simulink model "SimScape_PSFB_PCMC_HalfBridge_SRMode0"  (R2023b)
settings: Solver=VariableStepAuto  StartTime=0.0  StopTime=0.5  RelTol=1e-3
undefined symbols (not defined in the file): ADC_MaxCount, ADC_Vref, Gi_fb, L, Lm, n, Rload, Ro, Tcmpss, transformerCoupling
libraries: ee_lib x15, fl_lib x14, nesl_utility x9, simulink_extras x2, simulink x2, slpidlib x1
(part 1 of 2)
settings Model: Creator=a0485298  LastModifiedBy=a0485298

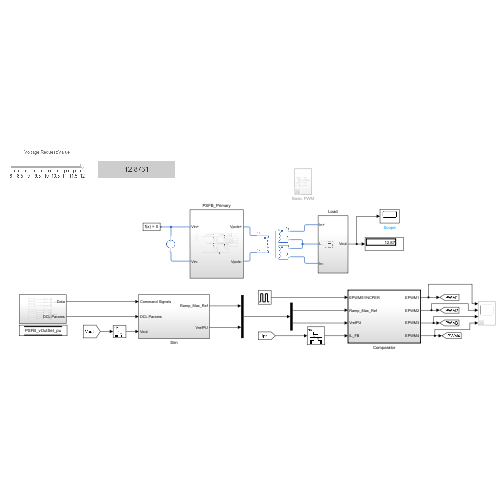
[thumbnail: Simulink's stored preview of the top-level diagram]
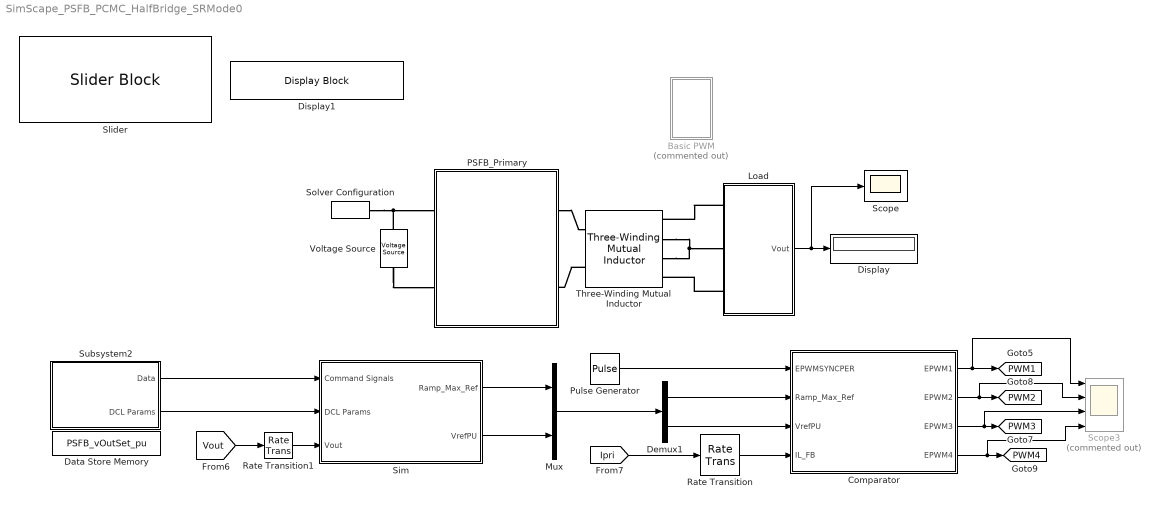
== system SimScape_PSFB_PCMC_HalfBridge_SRMode0 ==
  Basic PWM : Subsystem  Commented=on
  Comparator : Subsystem  TreatAsAtomicUnit=on
  Data Store Memory : DataStoreMemory  DataStoreName=PSFB_vOutSet_pu  WriteAfterWriteMsg=warning  ShowAdditionalParam=off
  Demux1 : Demux  Outputs=2
  Display : Display
  Display1 : DisplayBlock  LabelPosition=Hide  Transparency=1
  Load : Subsystem
      settings: PortSchema="{\"entries\":[{\"content\":{\"sides\":[{\"content\":{\"connectorIds\":[\"Out1\"]},\"type\":\"ConnectorPlacement.EquallySpacedRectSide\",\"uuid\":\"d456934f-8cdc-4057-8992-94e9047cf07f\"},{\"content\":{\"connectorIds\":[\"RConn1\",\"RConn2\",\"RConn3\"],\"side\":\"RIGHT\"},\"type\":\"ConnectorPlacement.EquallySpacedRectSide\",\"uuid\":\"13bc9f8f-848a-4da9-bcdd-c680aa1b8ed2\"},{\"content\":{\"side\":\"TOP\"},\"type\":\"ConnectorPlacement.EquallySpacedRectSide\",\"uuid\":\"cb883331-c911-4e56-96a8-3c5b8591d015\"}]},\"type\":\"ConnectorPlacement.EquallySpacedConnector\",\"uuid\":\"df461162-389f-468c-a658-0242576d1be7\"}],\"packageUris\":[\"http://schema.mathworks.com/mf0/Connector/R2020b\"],\"version\":\"1.0\"}"
  Mux : Mux  Inputs=2
  PSFB_Primary : Subsystem
  Pulse Generator : DiscretePulseGenerator  PulseType=Time based  Period=1/200e3  PulseWidth=5
  Rate Transition : RateTransition
  Rate Transition1 : RateTransition
  Scope : Scope
  Scope3 : Scope  Commented=on  NumInputPorts=4
  Sim : Subsystem  RTWFileName=sample_cla  VariantControl=(sim)
      settings: RTWSystemCode=Nonreusable function  RTWFileNameOpts=User specified  FunctionWithSeparateData=on  RTWMemSecFuncInitTerm=C28xFunction  RTWMemSecFuncExecute=ClaFunction  RTWMemSecDataConstants=Cla1DataRam  RTWMemSecDataInternal=Cla1DataRam  RTWMemSecDataParameters=Cla1DataRam
  Slider : SliderBlock  ScaleMin=8  ScaleMax=12  TickInterval=0.5
  Solver Configuration : nesl_utility/Solver Configuration  PhysicalDomain=network_engine_domain  SubClassName=solver  LeftPortType=input  RightPortType=generic  Tones=[]  Harmonics=[]  SimulateNoise=off  Profile=off  UseLocalSampling=off  EnableSwitchedLinearOptims=on  FrequencyDomain=off  UseCCode=off  RelTol=0.001  AbsTol=0.001  MinStep=1e-09  ToWorkspace=off  RevertToSquareIcSolve=off  NumHomotopyIterations=100  PhasorMode=off  PhasorModeNumHarmonics=1  ConsistencySolver=NEWTON_XTOL_AFTER_FTOL  IndexReductionMethod=DerivativeReplacement  DoDC=off  ResidualTolerance=1e-09  ConsistencyTolSource=GLOBAL  ConsistencyAbsTol=0.001  ConsistencyRelTol=0.001  ConsistencyTolFactor=0.001  UseLocalSolver=on  LocalSolverChoice=NE_BACKWARD_EULER_ADVANCER  ResolveIndetEquations=on  FunctionEvalNumThread=1  LocalSolverSampleTime=1/120e6  DoFixedCost=off  MaxNonlinIter=3  MaxModeIter=2  ComputeImpulses=off  ImpulseIterations=2  LinearAlgebra=auto  LinearAlgebraNumThread=0  EquationFormulation=NE_TIME_EF  DelaysMemoryBudget=1024  AutomaticFiltering=off  FilteringTimeConstant=0.001  PartitionStorageMethod=AS_NEEDED  PartitionMemoryBudget=1024  PartitionMethod=ROBUST  MultibodyUseLocalSolver=off  MultibodyLocalSolverChoice=ODE1  MultibodyLocalSolverSampleTime=0.001
  Subsystem2 : Subsystem
  Three-Winding Mutual Inductor : ee_lib/Passive/Transformers/Three-Winding Mutual Inductor  L1=Lm/transformerCoupling^2 H  L2=Lm/n^2 H  L3=Lm/n^2 H  K12=transformerCoupling  K13=transformerCoupling  K23=transformerCoupling  IC_given=1  IC1=0 A  IC2=0 A  IC3=0 A
      settings: InternalSimscapePortConfiguration="{\"Bottom\":[],\"Left\":[{\"id\":\"p1\",\"label\":\"1+\",\"type\":\"foundation.electrical.electrical\"},{\"id\":\"n1\",\"label\":\"1-\",\"type\":\"foundation.electrical.electrical\"}],\"Right\":[{\"id\":\"p2\",\"label\":\"2+\",\"type\":\"foundation.electrical.electrical\"},{\"id\":\"n2\",\"label\":\"2-\",\"type\":\"foundation.electrical.electrical\"},{\"id\":\"p3\",\"label\":\"3+\",\"type\":\"foundation.electrical.electrical\"},{\"id\":\"n3\",\"label\":\"3-\",\"type\":\"foundation.electrical.electrical\"}],\"Top\":[]}"
  Voltage Source : ee_lib/Sources/Voltage Source  dc_voltage=Vin V  ac_voltage=0 V  ac_shift=0 rad  ac_frequency=60 Hz  noise_mode=ee.enum.sources.noise.Disabled  PSD=0 V^2/Hz  sample_time=1e-3 s  repeatability=ee.enum.sources.repeatability.NotRepeatable  user_seed=0  auto_seed=3890346746  i_specify=off  i_priority=None  i=0 A  i_nominal_specify=off  i_nominal_unit=A  i_nominal_value=1  v_specify=off  v_priority=None  v=0 V  v_nominal_specify=off  v_nominal_unit=V  v_nominal_value=1
  tag scope: PWM1=global, PWM2=global, PWM3=global, PWM4=global
  wires:
  Load/1(Vout) -> Scope/1, Display/1
  Demux1/2 -> Comparator/3(VrefPU)
  Sim/1(Ramp_Max_Ref) -> Mux/1
  Mux/1 -> Demux1/1
  Comparator/2(EPWM2) -> Scope3/2, [PWM2]
  Subsystem2/2(DCL Params) -> Sim/2(DCL Params)
  [Vout] -> Rate Transition1/1
  Pulse Generator/1 -> Comparator/1(EPWMSYNCPER)
  Comparator/4(EPWM4) -> Scope3/4, [PWM4]
  Comparator/1(EPWM1) -> Scope3/1, [PWM1]
  Demux1/1 -> Comparator/2(Ramp_Max_Ref)
  Subsystem2/1(Data) -> Sim/1(Command Signals)
  Comparator/3(EPWM3) -> Scope3/3, [PWM3]
  Sim/2(VrefPU) -> Mux/2
  [Ipri] -> Rate Transition/1
  Rate Transition1/1 -> Sim/3(Vout)
  Rate Transition/1 -> Comparator/4(IL_FB)
  connections:
  Load/RConn3 -- Three-Winding Mutual Inductor/RConn4
  Three-Winding Mutual Inductor/RConn2 -- Three-Winding Mutual Inductor/RConn3 -- Load/RConn2
  Three-Winding Mutual Inductor/LConn2 -- PSFB_Primary/LConn2
  PSFB_Primary/LConn1 -- Three-Winding Mutual Inductor/LConn1
  Load/RConn1 -- Three-Winding Mutual Inductor/RConn1
  Voltage Source/LConn1 -- PSFB_Primary/RConn1 -- Solver Configuration/RConn1
  Voltage Source/RConn1 -- PSFB_Primary/RConn2

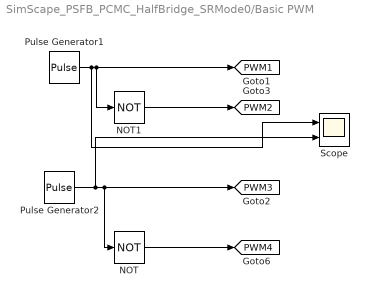
== system SimScape_PSFB_PCMC_HalfBridge_SRMode0/Basic PWM ==
  NOT : Logic  Operator=NOT  IconShape=distinctive  AllPortsSameDT=off  OutDataTypeStr=boolean
  NOT1 : Logic  Operator=NOT  IconShape=distinctive  AllPortsSameDT=off  OutDataTypeStr=boolean
  Pulse Generator1 : DiscretePulseGenerator  PulseType=Time based  Period=1/100e3  PulseWidth=50
  Pulse Generator2 : DiscretePulseGenerator  PulseType=Time based  Period=1/100e3  PulseWidth=50  PhaseDelay=(72/(180*100e3))
  Scope : Scope  NumInputPorts=2
  tag scope: PWM1=global, PWM2=global, PWM3=global, PWM4=global
  wires:
  Pulse Generator1/1 -> Scope/1, [PWM1], NOT1/1
  NOT1/1 -> [PWM2]
  Pulse Generator2/1 -> Scope/2, [PWM3], NOT/1
  NOT/1 -> [PWM4]

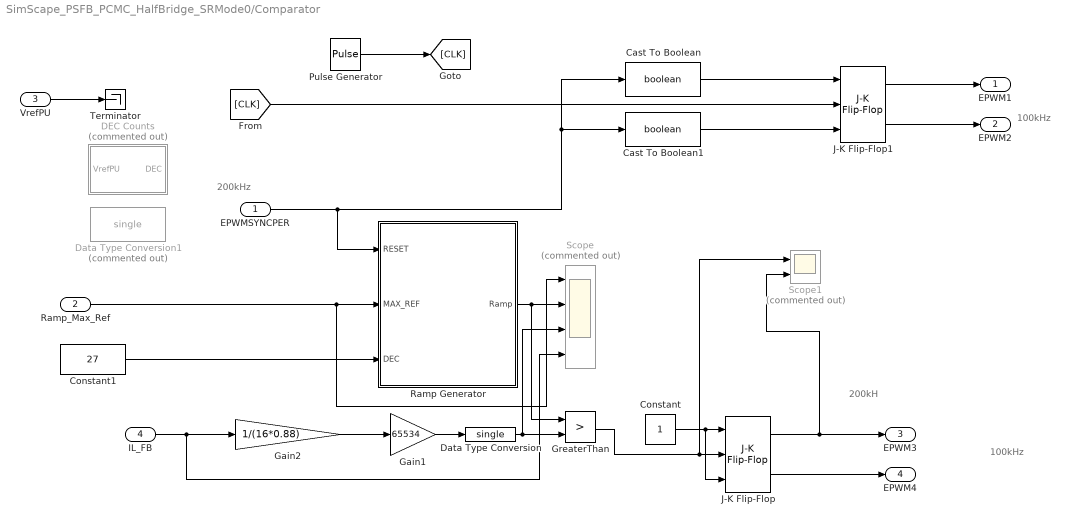
== system SimScape_PSFB_PCMC_HalfBridge_SRMode0/Comparator ==
  note: 200kH
  note: 100kHz
  note: 100kHz
  note: 200kHz
  EPWMSYNCPER : Inport
  Ramp_Max_Ref : Inport  Port=2
  VrefPU : Inport  Port=3
  IL_FB : Inport  Port=4
  Cast To Boolean : DataTypeConversion  OutDataTypeStr=boolean  SaturateOnIntegerOverflow=off  RndMeth=Floor
  Cast To Boolean1 : DataTypeConversion  OutDataTypeStr=boolean  SaturateOnIntegerOverflow=off  RndMeth=Floor
  Constant : Constant  OutDataTypeStr=boolean
  Constant1 : Constant  Value=27  OutDataTypeStr=single
  DEC Counts : Subsystem  Commented=on
  Data Type Conversion : DataTypeConversion  OutDataTypeStr=single  SaturateOnIntegerOverflow=off  RndMeth=Floor
  Data Type Conversion1 : DataTypeConversion  Commented=on  OutDataTypeStr=single  SaturateOnIntegerOverflow=off  RndMeth=Floor
  Gain1 : Gain  Gain=65534  OutDataTypeStr=single
  Gain2 : Gain  Gain=1/(16*0.88)  OutDataTypeStr=single
  GreaterThan : RelationalOperator  Operator=>  OutDataTypeStr=boolean  RndMeth=Simplest  InputSameDT=off
  J-K Flip-Flop : simulink_extras/Flip Flops/J-K Flip-Flop  initial_condition=0
  J-K Flip-Flop1 : simulink_extras/Flip Flops/J-K Flip-Flop  initial_condition=0
  Pulse Generator : DiscretePulseGenerator  PulseType=Time based  Period=1/(2*200e3)
  Ramp Generator : Subsystem
  Scope : Scope  Commented=on  NumInputPorts=4
  Scope1 : Scope  Commented=on  NumInputPorts=2
  Terminator : Terminator
  EPWM1 : Outport
  EPWM2 : Outport  Port=2
  EPWM3 : Outport  Port=3
  EPWM4 : Outport  Port=4
  wires:
  Gain2/1 -> Gain1/1
  IL_FB/1 -> Scope/4, Gain2/1
  EPWMSYNCPER/1 -> Cast To Boolean1/1, Cast To Boolean/1, Ramp Generator/1(RESET)
  Ramp Generator/1(Ramp) -> GreaterThan/1, Scope/2
  Gain1/1 -> Data Type Conversion/1
  J-K Flip-Flop/1 -> Scope1/2, EPWM3/1
  J-K Flip-Flop/2 -> EPWM4/1
  Pulse Generator/1 -> [CLK]
  [CLK] -> J-K Flip-Flop1/2
  J-K Flip-Flop1/1 -> EPWM1/1
  J-K Flip-Flop1/2 -> EPWM2/1
  Cast To Boolean/1 -> J-K Flip-Flop1/1
  Cast To Boolean1/1 -> J-K Flip-Flop1/3
  VrefPU/1 -> Terminator/1
  Constant1/1 -> Ramp Generator/3(DEC)
  Constant/1 -> J-K Flip-Flop/3, J-K Flip-Flop/1
  GreaterThan/1 -> Scope1/1, J-K Flip-Flop/2
  Ramp_Max_Ref/1 -> Scope/1, Ramp Generator/2(MAX_REF)
  Data Type Conversion/1 -> Scope/3, GreaterThan/2

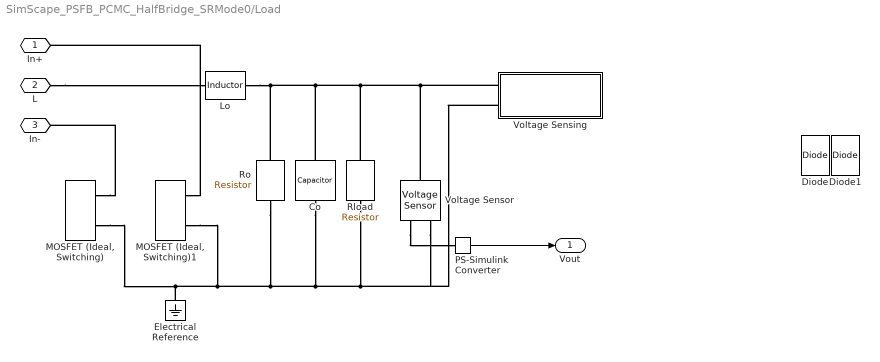
== system SimScape_PSFB_PCMC_HalfBridge_SRMode0/Load ==
  Co : fl_lib/Electrical/Electrical Elements/Capacitor  c=Co F  r=1e-6 Ohm  g=0 1/Ohm  i_specify=off  i_priority=None  i=0 A  i_nominal_specify=off  i_nominal_unit=A  i_nominal_value=1  v_specify=off  v_priority=None  v=0 V  v_nominal_specify=off  v_nominal_unit=V  v_nominal_value=30  vc_specify=off  vc_priority=High  vc=0 V  vc_nominal_specify=off  vc_nominal_unit=V  vc_nominal_value=1
  Diode : ee_lib/Semiconductors & Converters/Diode  ModelType=ee.enum.diode.modelType.pwl  TableType=ee.enum.diode.tableType.IfMat  IfMat=[.07, .12, .19, 1.75, 4.24, 7.32, 11.2; .16, .3, .72, 2.14, 5.02, 8.35, 13.12] A  VfMat=[.9, 1.15, 1.25, 1.5, 1.75, 2.17, 2.6, 2.85; .58, .68, .75, 1.1, 1.38, 1.77, 2.27, 2.7] V  TjVec=[25, 125] degC  VfVec=[.5, .7, .9, 1.3, 1.7, 2.1, 2.5] V  IfVec=[.1, .2, .5, 1, 2, 4, 7, 10] A  Vf=0.6 V  Ron=1e-6 Ohm  Goff=1e-8 S  prmExp=ee.enum.diode.expParam.useTwo  I12=[.0137, .545] A  V12=[.6, .7] V  RS=0 Ohm  Tmeas=25 degC  IS=1e-12 A  ec=1  I1=0.0137 A  V1=0.6 V  N_series=1  N_parallel=1  ZenerEnable=false  Rz=0.3 Ohm  BV=inf V  C_param=ee.enum.diode.capParam.fixed  CJ=0 pF  CJ0=5 pF  Vvec=[.1, 10, 100] V  Cvec=[3.5, 1, .4] pF  VJ=1 V  Mgrad=0.5  FC=0.5  Q_param=ee.enum.diode.recoveryParam.off  iRM=-7.15 A  iF=4 A  didt=-750 A/us  trr_factor=3  trr=115 ns  Qrr=150 nA*s  Vr=-600 V  Ls=150 nH  Erec=0.03 J  TT=50 ns  tau=100 ns  T_param=ee.enum.diode.temperatureParam.off  Tdevice=25 degC  I1_T2=0.245 A  V1_T2=0.5 V  IS_T2=1.25e-7 A  Tmeas2=125 degC  XTI_param=ee.enum.diode.xtiParam.pn  XTI=3  EG_param=ee.enum.diode.egapParam.material_si  EG=1.11 eV  dBVdT=0 V/K  enable_faults=simscape.enum.onoff.off  fault_action=simscape.enum.assert.action.none  fault_types=ee.enum.diode.faults.open  tau_fault=1e-3 s  IfMat_faulted=[.07, .12, .19, 1.75, 4.24, 7.32, 11.2; .16, .3, .72, 2.14, 4.02, 6.35, 9.12] A  VfMat_faulted=[.9, 1.15, 1.25, 1.5, 1.75, 2.17, 2.6, 2.85; .58, .68, .75, 1.1, 1.38, 1.77, 2.27, 2.7] V  VfVec_faulted=[.5, .7, .9, 1.3, 1.7, 2.1, 2.5] V  IfVec_faulted=[.1, .2, .5, 1, 2, 4, 7, 10] A  Ropen_faulted=1000 Ohm  Gshort_faulted=1000 1/Ohm  Vf_faulted=0.6 V  Ron_faulted=0.3 Ohm  Goff_faulted=1e-8 S  I12_faulted=[.0137, .545] A  V12_faulted=[.6, .7] V  IS_faulted=1e-12 A  ec_faulted=1  I1_faulted=0.0137 A  V1_faulted=0.6 V  RS_faulted=0 Ohm  Rz_faulted=0.3 Ohm  BV_faulted=inf V  Cscale_faulted=100  fault_trigger=ee.enum.faults.faultTrigger.temporal  t_fault=inf s  max_permissible_voltage=inf V  n_fail_on_voltage=1  max_permissible_current=inf A  t_fail_on_current=1 s  max_permissible_dVdt=inf V/s  enable_fault_input=simscape.enum.onoff.off  i_specify=off  i_priority=None  i=0 A  i_nominal_specify=off  i_nominal_unit=A  i_nominal_value=1  v_specify=off  v_priority=None  v=0 V  v_nominal_specify=off  v_nominal_unit=V  v_nominal_value=1  v_capacitor_specify=off  v_capacitor_priority=None  v_capacitor=0 V  v_capacitor_nominal_specify=off  v_capacitor_nominal_unit=V  v_capacitor_nominal_value=1  faulted_specify=off  faulted_priority=None  faulted=0  faulted_nominal_specify=off  faulted_nominal_unit=1  faulted_nominal_value=1  i_diode_specify=off  i_diode_priority=None  i_diode=0 A  i_diode_nominal_specify=off  i_diode_nominal_unit=A  i_diode_nominal_value=1  v_diode_specify=off  v_diode_priority=None  v_diode=0 V  v_diode_nominal_specify=off  v_diode_nominal_unit=V  v_diode_nominal_value=1  i_capacitor_specify=off  i_capacitor_priority=None  i_capacitor=0 A  i_capacitor_nominal_specify=off  i_capacitor_nominal_unit=A  i_capacitor_nominal_value=1  power_dissipated_specify=off  power_dissipated_priority=None  power_dissipated=0 W  power_dissipated_nominal_specify=off  power_dissipated_nominal_unit=W  power_dissipated_nominal_value=1  fidelity_level=ee.enum.diode.fidelity.includeChargeDyn  rec_loss_model=ee.enum.diode.reverseRecoveryModel.fixed  ErecVal=0 J  scaleWithIandV=true  ErecMat=zeros(2, 3) J  TjrecVec=[298.15, 398.15] K  IfrecVec=[.1, 1, 10] A  IrecVal=10 A  VrecVal=10 V  tFilter=1 / 1000 / 100 s  max_permissible_temperature=inf K  t_fail_on_temperature=1 s  thermal_network_parameterization=ee.enum.thermalNetworkTopology.junctionCase  Rth=[0, 10] K/W  Rth_Cauer=[1, 3, 10] K/W  Rth_Foster=[4, 6] K/W  thermal_mass_parameterization=ee.enum.thermalNetwork.timeconstant  thermal_mass=[0, 1] J/K  thermal_mass_Cauer=[.1, .3, 1] J/K  thermal_mass_Foster=[1.5, 3] J/K  thermal_time_constant=[0, 10] s  thermal_time_constant_Cauer=[1, 3, 10] s  thermal_time_constant_Foster=[6, 18] s  thermal_mass_initial_temperatures=[25, 25] degC  thermal_mass_initial_temperatures_Cauer=[25, 25, 25] degC  junction_thermal_mass=0.01 J/K  Tvec_initial_Foster=[25, 25, 25, 25] degC  no_thermal_network=0  junction_temperature_specify=off  junction_temperature_priority=None  junction_temperature=25 degC  junction_temperature_nominal_specify=off  junction_temperature_nominal_unit=degC  junction_temperature_nominal_value=1
  Diode1 : ee_lib/Semiconductors & Converters/Diode  ModelType=ee.enum.diode.modelType.pwl  TableType=ee.enum.diode.tableType.IfMat  IfMat=[.07, .12, .19, 1.75, 4.24, 7.32, 11.2; .16, .3, .72, 2.14, 5.02, 8.35, 13.12] A  VfMat=[.9, 1.15, 1.25, 1.5, 1.75, 2.17, 2.6, 2.85; .58, .68, .75, 1.1, 1.38, 1.77, 2.27, 2.7] V  TjVec=[25, 125] degC  VfVec=[.5, .7, .9, 1.3, 1.7, 2.1, 2.5] V  IfVec=[.1, .2, .5, 1, 2, 4, 7, 10] A  Vf=0.6 V  Ron=1e-6 Ohm  Goff=1e-8 S  prmExp=ee.enum.diode.expParam.useTwo  I12=[.0137, .545] A  V12=[.6, .7] V  RS=0 Ohm  Tmeas=25 degC  IS=1e-12 A  ec=1  I1=0.0137 A  V1=0.6 V  N_series=1  N_parallel=1  ZenerEnable=false  Rz=0.3 Ohm  BV=inf V  C_param=ee.enum.diode.capParam.fixed  CJ=0 pF  CJ0=5 pF  Vvec=[.1, 10, 100] V  Cvec=[3.5, 1, .4] pF  VJ=1 V  Mgrad=0.5  FC=0.5  Q_param=ee.enum.diode.recoveryParam.off  iRM=-7.15 A  iF=4 A  didt=-750 A/us  trr_factor=3  trr=115 ns  Qrr=150 nA*s  Vr=-600 V  Ls=150 nH  Erec=0.03 J  TT=50 ns  tau=100 ns  T_param=ee.enum.diode.temperatureParam.off  Tdevice=25 degC  I1_T2=0.245 A  V1_T2=0.5 V  IS_T2=1.25e-7 A  Tmeas2=125 degC  XTI_param=ee.enum.diode.xtiParam.pn  XTI=3  EG_param=ee.enum.diode.egapParam.material_si  EG=1.11 eV  dBVdT=0 V/K  enable_faults=simscape.enum.onoff.off  fault_action=simscape.enum.assert.action.none  fault_types=ee.enum.diode.faults.open  tau_fault=1e-3 s  IfMat_faulted=[.07, .12, .19, 1.75, 4.24, 7.32, 11.2; .16, .3, .72, 2.14, 4.02, 6.35, 9.12] A  VfMat_faulted=[.9, 1.15, 1.25, 1.5, 1.75, 2.17, 2.6, 2.85; .58, .68, .75, 1.1, 1.38, 1.77, 2.27, 2.7] V  VfVec_faulted=[.5, .7, .9, 1.3, 1.7, 2.1, 2.5] V  IfVec_faulted=[.1, .2, .5, 1, 2, 4, 7, 10] A  Ropen_faulted=1000 Ohm  Gshort_faulted=1000 1/Ohm  Vf_faulted=0.6 V  Ron_faulted=0.3 Ohm  Goff_faulted=1e-8 S  I12_faulted=[.0137, .545] A  V12_faulted=[.6, .7] V  IS_faulted=1e-12 A  ec_faulted=1  I1_faulted=0.0137 A  V1_faulted=0.6 V  RS_faulted=0 Ohm  Rz_faulted=0.3 Ohm  BV_faulted=inf V  Cscale_faulted=100  fault_trigger=ee.enum.faults.faultTrigger.temporal  t_fault=inf s  max_permissible_voltage=inf V  n_fail_on_voltage=1  max_permissible_current=inf A  t_fail_on_current=1 s  max_permissible_dVdt=inf V/s  enable_fault_input=simscape.enum.onoff.off  i_specify=off  i_priority=None  i=0 A  i_nominal_specify=off  i_nominal_unit=A  i_nominal_value=1  v_specify=off  v_priority=None  v=0 V  v_nominal_specify=off  v_nominal_unit=V  v_nominal_value=1  v_capacitor_specify=off  v_capacitor_priority=None  v_capacitor=0 V  v_capacitor_nominal_specify=off  v_capacitor_nominal_unit=V  v_capacitor_nominal_value=1  faulted_specify=off  faulted_priority=None  faulted=0  faulted_nominal_specify=off  faulted_nominal_unit=1  faulted_nominal_value=1  i_diode_specify=off  i_diode_priority=None  i_diode=0 A  i_diode_nominal_specify=off  i_diode_nominal_unit=A  i_diode_nominal_value=1  v_diode_specify=off  v_diode_priority=None  v_diode=0 V  v_diode_nominal_specify=off  v_diode_nominal_unit=V  v_diode_nominal_value=1  i_capacitor_specify=off  i_capacitor_priority=None  i_capacitor=0 A  i_capacitor_nominal_specify=off  i_capacitor_nominal_unit=A  i_capacitor_nominal_value=1  power_dissipated_specify=off  power_dissipated_priority=None  power_dissipated=0 W  power_dissipated_nominal_specify=off  power_dissipated_nominal_unit=W  power_dissipated_nominal_value=1  fidelity_level=ee.enum.diode.fidelity.includeChargeDyn  rec_loss_model=ee.enum.diode.reverseRecoveryModel.fixed  ErecVal=0 J  scaleWithIandV=true  ErecMat=zeros(2, 3) J  TjrecVec=[298.15, 398.15] K  IfrecVec=[.1, 1, 10] A  IrecVal=10 A  VrecVal=10 V  tFilter=1 / 1000 / 100 s  max_permissible_temperature=inf K  t_fail_on_temperature=1 s  thermal_network_parameterization=ee.enum.thermalNetworkTopology.junctionCase  Rth=[0, 10] K/W  Rth_Cauer=[1, 3, 10] K/W  Rth_Foster=[4, 6] K/W  thermal_mass_parameterization=ee.enum.thermalNetwork.timeconstant  thermal_mass=[0, 1] J/K  thermal_mass_Cauer=[.1, .3, 1] J/K  thermal_mass_Foster=[1.5, 3] J/K  thermal_time_constant=[0, 10] s  thermal_time_constant_Cauer=[1, 3, 10] s  thermal_time_constant_Foster=[6, 18] s  thermal_mass_initial_temperatures=[25, 25] degC  thermal_mass_initial_temperatures_Cauer=[25, 25, 25] degC  junction_thermal_mass=0.01 J/K  Tvec_initial_Foster=[25, 25, 25, 25] degC  no_thermal_network=0  junction_temperature_specify=off  junction_temperature_priority=None  junction_temperature=25 degC  junction_temperature_nominal_specify=off  junction_temperature_nominal_unit=degC  junction_temperature_nominal_value=1
  Electrical Reference : fl_lib/Electrical/Electrical Elements/Electrical Reference
  Lo : ee_lib/Passive/Inductor  l=Lo H  enable_L_tol=ee.enum.toleranceApplication.none  L_tol=20  tol_distribution=ee.enum.toleranceDistribution.uniform  nSigma=4  r=0 Ohm  g=1e-9 1/Ohm  enable_operating_limits=ee.enum.enable.no  operating_limit_action=ee.enum.passive.reportOpLim.warn  max_working_current=1 A  power_rating=1 W  enable_faults=ee.enum.enable.no  fault_action=simscape.enum.assert.action.none  lambdaPercent=50  k_faulted=0.9999  turnsShort=ee.enum.passive.inductor.turnsShortOption.no  openCct=ee.enum.enable.no  groundShort=ee.enum.passive.inductor.groundShortOption.no  groundShortG=0 1/Ohm  tau_fault=1e-3 s  fault_trigger=ee.enum.faults.faultTrigger.temporal  t_fault=1 s  max_permissible_voltage=100 V  n_fail_on_voltage=1  max_permissible_current=1 A  t_fail_on_current=1 s  i_L_specify=off  i_L_priority=High  i_L=0 A  i_L_nominal_specify=off  i_L_nominal_unit=A  i_L_nominal_value=1
  "MOSFET (Ideal, Switching)" : ee_lib/Semiconductors & Converters/MOSFET (Ideal, Switching)  port_option=ee.enum.controlport.ps  Rds=0.01 Ohm  Goff=1e-6 1/Ohm  Vth=2 V  diode_param=ee.enum.converters.protectiondiode.nodynamics  diode_Vf=0.8 V  diode_Ron=0.001 Ohm  diode_Goff=1e-5 1/Ohm  diode_C=50e-9 F  diode_iRM=-235 A  diode_iF=300 A  diode_idot=-50 A/us  diode_trr_param=ee.enum.converters.diodeReverseParam.trr_factor  diode_trr_factor=3  diode_trr=15 us  diode_Qrr=1500 s*uA  ids_specify=off  ids_priority=None  ids=0 A  ids_nominal_specify=off  ids_nominal_unit=A  ids_nominal_value=1  vds_specify=off  vds_priority=None  vds=0 V  vds_nominal_specify=off  vds_nominal_unit=V  vds_nominal_value=1  vgs_specify=off  vgs_priority=None  vgs=0 V  vgs_nominal_specify=off  vgs_nominal_unit=V  vgs_nominal_value=1  thermal_loss_option=ee.enum.converters.thermalLossOption.constantvalues  Von_data=[0, 1.8, 3.2, 6, 10, 16; 0, 2, 5.5, 9.5, 15, 25] V  Tj=[298.15, 448.15] K  Iout_data=[0, 20, 40, 60, 80, 100] A  Eon_data=[0, 55.04, 124.57, 235.53, 362.12; 0, 71.25, 161.25, 304.88, 468.75] * 1e-6 J  Eoff_data=[0, 18, 30, 56.1, 76.5; 0, 22.5, 37.5, 70.13, 95.63] * 1e-6 J  Eon_data_3D=[zeros(2, 5, 3)] J  Eoff_data_3D=[zeros(2, 5, 3)] J  Tj_loss=[298.15, 448.15] K  Iout_data_loss=[0, 10, 20, 30, 40] A  tabulateWithVds=false  Vds_loss=[0, 150, 300] V  Eon_scalar=22.86e-3 J  Eoff_scalar=17.14e-3 J  Voff=300 V  Iout_scalar=600 A  useCurrentFromPreviousCycle=false  useVoltageFromPreviousCycle=false  diodeModelType=ee.enum.converters.diodeModelType.pwl  diodeTableType=ee.enum.diode.tableType.IfMat  diode_IfMat=[.07, .12, .19, 1.75, 4.24, 7.32, 11.2; .16, .3, .72, 2.14, 4.02, 6.35, 9.12] A  diode_VfMat=[.9, 1.15, 1.25, 1.5, 1.75, 2.17, 2.6, 2.85; .58, .68, .75, 1.1, 1.38, 1.77, 2.27, 2.7] V  diode_TjVec=[25, 125] degC  diode_VfVec=[.5, .7, .9, 1.3, 1.7, 2.1, 2.5] V  diode_IfVec=[.1, .2, .5, 1, 2, 4, 7, 10] A  diode_Vr=-600 V  diode_Ls=150 nH  diode_Erec=0.03 J  diode_rec_loss_model=ee.enum.diode.reverseRecoveryModel.fixed  diode_ErecVal=0 J  diode_scaleWithIandV=true  diode_ErecMat=zeros(2, 3) J  diode_TjrecVec=[298.15, 398.15] K  diode_IfrecVec=[.1, 1, 10] A  diode_IrecVal=10 A  diode_VrecVal=10 V  diode_tFilter=1 / 1000 / 100 s  thermal_network_parameterization=ee.enum.thermalNetworkTopology.external  Rth=[.03, .2] K/W  Rth_Cauer=[.03, .1, .2] K/W  Rth_Foster=[.03, .2] K/W  thermal_mass_parameterization=ee.enum.thermalNetwork.timeconstant  thermal_mass=[3, 25] J/K  thermal_mass_Cauer=[3, 10, 25] J/K  thermal_mass_Foster=[33, 50] J/K  thermal_time_constant=[.1, 5] s  thermal_time_constant_Cauer=[.1, 1, 5] s  thermal_time_constant_Foster=[1, 10] s  thermal_mass_initial_temperatures=[25, 25] degC  thermal_mass_initial_temperatures_Cauer=[25, 25, 25] degC  junction_thermal_mass=0.1 J/K  Tvec_initial_Foster=[25, 25, 25, 25] degC  no_thermal_network=0  junction_temperature_specify=off  junction_temperature_priority=None  junction_temperature=25 degC  junction_temperature_nominal_specify=off  junction_temperature_nominal_unit=degC  junction_temperature_nominal_value=1  Qj_specify=off  Qj_priority=None  Qj=0 W  Qj_nominal_specify=off  Qj_nominal_unit=W  Qj_nominal_value=1  accumulatedSwitchingLosses_specify=off  accumulatedSwitchingLosses_priority=None  accumulatedSwitchingLosses=0 J
  "MOSFET (Ideal, Switching)1" : ee_lib/Semiconductors & Converters/MOSFET (Ideal, Switching)  port_option=ee.enum.controlport.ps  Rds=0.01 Ohm  Goff=1e-6 1/Ohm  Vth=2 V  diode_param=ee.enum.converters.protectiondiode.nodynamics  diode_Vf=0.8 V  diode_Ron=0.001 Ohm  diode_Goff=1e-5 1/Ohm  diode_C=50e-9 F  diode_iRM=-235 A  diode_iF=300 A  diode_idot=-50 A/us  diode_trr_param=ee.enum.converters.diodeReverseParam.trr_factor  diode_trr_factor=3  diode_trr=15 us  diode_Qrr=1500 s*uA  ids_specify=off  ids_priority=None  ids=0 A  ids_nominal_specify=off  ids_nominal_unit=A  ids_nominal_value=1  vds_specify=off  vds_priority=None  vds=0 V  vds_nominal_specify=off  vds_nominal_unit=V  vds_nominal_value=1  vgs_specify=off  vgs_priority=None  vgs=0 V  vgs_nominal_specify=off  vgs_nominal_unit=V  vgs_nominal_value=1  thermal_loss_option=ee.enum.converters.thermalLossOption.constantvalues  Von_data=[0, 1.8, 3.2, 6, 10, 16; 0, 2, 5.5, 9.5, 15, 25] V  Tj=[298.15, 448.15] K  Iout_data=[0, 20, 40, 60, 80, 100] A  Eon_data=[0, 55.04, 124.57, 235.53, 362.12; 0, 71.25, 161.25, 304.88, 468.75] * 1e-6 J  Eoff_data=[0, 18, 30, 56.1, 76.5; 0, 22.5, 37.5, 70.13, 95.63] * 1e-6 J  Eon_data_3D=[zeros(2, 5, 3)] J  Eoff_data_3D=[zeros(2, 5, 3)] J  Tj_loss=[298.15, 448.15] K  Iout_data_loss=[0, 10, 20, 30, 40] A  tabulateWithVds=false  Vds_loss=[0, 150, 300] V  Eon_scalar=22.86e-3 J  Eoff_scalar=17.14e-3 J  Voff=300 V  Iout_scalar=600 A  useCurrentFromPreviousCycle=false  useVoltageFromPreviousCycle=false  diodeModelType=ee.enum.converters.diodeModelType.pwl  diodeTableType=ee.enum.diode.tableType.IfMat  diode_IfMat=[.07, .12, .19, 1.75, 4.24, 7.32, 11.2; .16, .3, .72, 2.14, 4.02, 6.35, 9.12] A  diode_VfMat=[.9, 1.15, 1.25, 1.5, 1.75, 2.17, 2.6, 2.85; .58, .68, .75, 1.1, 1.38, 1.77, 2.27, 2.7] V  diode_TjVec=[25, 125] degC  diode_VfVec=[.5, .7, .9, 1.3, 1.7, 2.1, 2.5] V  diode_IfVec=[.1, .2, .5, 1, 2, 4, 7, 10] A  diode_Vr=-600 V  diode_Ls=150 nH  diode_Erec=0.03 J  diode_rec_loss_model=ee.enum.diode.reverseRecoveryModel.fixed  diode_ErecVal=0 J  diode_scaleWithIandV=true  diode_ErecMat=zeros(2, 3) J  diode_TjrecVec=[298.15, 398.15] K  diode_IfrecVec=[.1, 1, 10] A  diode_IrecVal=10 A  diode_VrecVal=10 V  diode_tFilter=1 / 1000 / 100 s  thermal_network_parameterization=ee.enum.thermalNetworkTopology.external  Rth=[.03, .2] K/W  Rth_Cauer=[.03, .1, .2] K/W  Rth_Foster=[.03, .2] K/W  thermal_mass_parameterization=ee.enum.thermalNetwork.timeconstant  thermal_mass=[3, 25] J/K  thermal_mass_Cauer=[3, 10, 25] J/K  thermal_mass_Foster=[33, 50] J/K  thermal_time_constant=[.1, 5] s  thermal_time_constant_Cauer=[.1, 1, 5] s  thermal_time_constant_Foster=[1, 10] s  thermal_mass_initial_temperatures=[25, 25] degC  thermal_mass_initial_temperatures_Cauer=[25, 25, 25] degC  junction_thermal_mass=0.1 J/K  Tvec_initial_Foster=[25, 25, 25, 25] degC  no_thermal_network=0  junction_temperature_specify=off  junction_temperature_priority=None  junction_temperature=25 degC  junction_temperature_nominal_specify=off  junction_temperature_nominal_unit=degC  junction_temperature_nominal_value=1  Qj_specify=off  Qj_priority=None  Qj=0 W  Qj_nominal_specify=off  Qj_nominal_unit=W  Qj_nominal_value=1  accumulatedSwitchingLosses_specify=off  accumulatedSwitchingLosses_priority=None  accumulatedSwitchingLosses=0 J
  PS-Simulink Converter : nesl_utility/PS-Simulink Converter  PhysicalDomain=network_engine_domain  SubClassName=ps_output  LeftPortType=input  RightPortType=output  PseudoPeriodic=off  Frequencies=[]  VectorFormat=inherit  Unit=inherit  AffineConversion=off
  Rload : fl_lib/Electrical/Electrical Elements/Resistor  R=Rload Ohm  i_specify=off  i_priority=None  i=0 A  i_nominal_specify=off  i_nominal_unit=A  i_nominal_value=1  v_specify=off  v_priority=None  v=0 V  v_nominal_specify=off  v_nominal_unit=V  v_nominal_value=1
  Ro : fl_lib/Electrical/Electrical Elements/Resistor  R=Ro/2 Ohm  i_specify=off  i_priority=None  i=0 A  i_nominal_specify=off  i_nominal_unit=A  i_nominal_value=1  v_specify=off  v_priority=None  v=0 V  v_nominal_specify=off  v_nominal_unit=V  v_nominal_value=1
  Voltage Sensing : Subsystem
  Voltage Sensor : fl_lib/Electrical/Electrical Sensors/Voltage Sensor
  In+ : PMIOPort  Side=Right
  L : PMIOPort  Port=2  Side=Right
  In- : PMIOPort  Port=3  Side=Right
  Vout : Outport
  wires:
  PS-Simulink Converter/1 -> Vout/1
  connections:
  Rload/RConn1 -- "MOSFET (Ideal, Switching)"/RConn2 -- Electrical Reference/LConn1 -- "MOSFET (Ideal, Switching)1"/RConn2 -- Ro/RConn1 -- Co/RConn1 -- Voltage Sensing/LConn2 -- Voltage Sensor/RConn2
  "MOSFET (Ideal, Switching)1"/RConn1 -- In+/RConn1
  "MOSFET (Ideal, Switching)"/RConn1 -- In-/RConn1
  Voltage Sensor/RConn1 -- PS-Simulink Converter/LConn1
  L/RConn1 -- Lo/LConn1
  Voltage Sensor/LConn1 -- Lo/RConn1 -- Ro/LConn1 -- Co/LConn1 -- Rload/LConn1 -- Voltage Sensing/LConn1

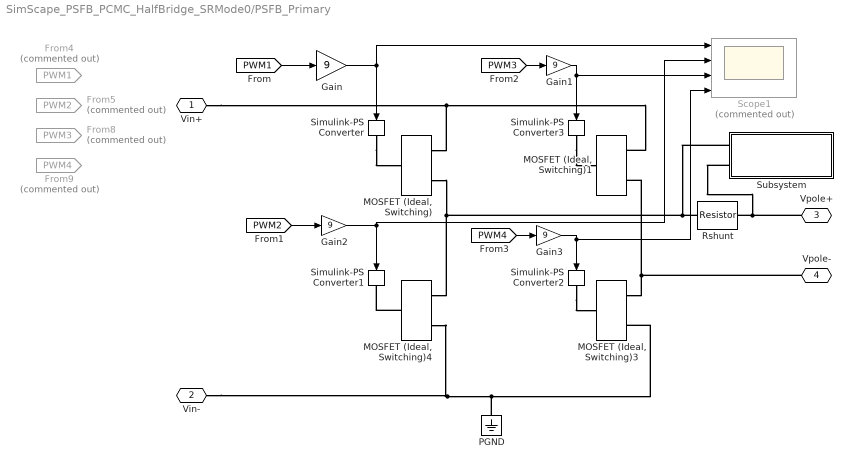
== system SimScape_PSFB_PCMC_HalfBridge_SRMode0/PSFB_Primary ==
  From4 : From  Commented=on  GotoTag=PWM1  TagVisibility=global
  From5 : From  Commented=on  GotoTag=PWM2  TagVisibility=global
  From8 : From  Commented=on  GotoTag=PWM3  TagVisibility=global
  From9 : From  Commented=on  GotoTag=PWM4  TagVisibility=global
  Gain{,1..3} (4 alike) : Gain  Gain=9  OutDataTypeStr=double
  MOSFET (Ideal, Switching){,1,3..4} (4 alike) : ee_lib/Semiconductors & Converters/MOSFET (Ideal, Switching)  port_option=ee.enum.controlport.ps  Rds=0.01 Ohm  Goff=1e-6 1/Ohm  Vth=2 V  diode_param=ee.enum.converters.protectiondiode.none  diode_Vf=0.8 V  diode_Ron=0.001 Ohm  diode_Goff=1e-5 1/Ohm  diode_C=50e-9 F  diode_iRM=-235 A  diode_iF=300 A  diode_idot=-50 A/us  diode_trr_param=ee.enum.converters.diodeReverseParam.trr_factor  diode_trr_factor=3  diode_trr=15 us  diode_Qrr=1500 s*uA  ids_specify=off  ids_priority=None  ids=0 A  ids_nominal_specify=off  ids_nominal_unit=A  ids_nominal_value=1  vds_specify=off  vds_priority=None  vds=0 V  vds_nominal_specify=off  vds_nominal_unit=V  vds_nominal_value=1  vgs_specify=off  vgs_priority=None  vgs=0 V  vgs_nominal_specify=off  vgs_nominal_unit=V  vgs_nominal_value=1  thermal_loss_option=ee.enum.converters.thermalLossOption.constantvalues  Von_data=[0, 1.8, 3.2, 6, 10, 16; 0, 2, 5.5, 9.5, 15, 25] V  Tj=[298.15, 448.15] K  Iout_data=[0, 20, 40, 60, 80, 100] A  Eon_data=[0, 55.04, 124.57, 235.53, 362.12; 0, 71.25, 161.25, 304.88, 468.75] * 1e-6 J  Eoff_data=[0, 18, 30, 56.1, 76.5; 0, 22.5, 37.5, 70.13, 95.63] * 1e-6 J  Eon_data_3D=[zeros(2, 5, 3)] J  Eoff_data_3D=[zeros(2, 5, 3)] J  Tj_loss=[298.15, 448.15] K  Iout_data_loss=[0, 10, 20, 30, 40] A  tabulateWithVds=false  Vds_loss=[0, 150, 300] V  Eon_scalar=22.86e-3 J  Eoff_scalar=17.14e-3 J  Voff=300 V  Iout_scalar=600 A  useCurrentFromPreviousCycle=false  useVoltageFromPreviousCycle=false  diodeModelType=ee.enum.converters.diodeModelType.pwl  diodeTableType=ee.enum.diode.tableType.IfMat  diode_IfMat=[.07, .12, .19, 1.75, 4.24, 7.32, 11.2; .16, .3, .72, 2.14, 4.02, 6.35, 9.12] A  diode_VfMat=[.9, 1.15, 1.25, 1.5, 1.75, 2.17, 2.6, 2.85; .58, .68, .75, 1.1, 1.38, 1.77, 2.27, 2.7] V  diode_TjVec=[25, 125] degC  diode_VfVec=[.5, .7, .9, 1.3, 1.7, 2.1, 2.5] V  diode_IfVec=[.1, .2, .5, 1, 2, 4, 7, 10] A  diode_Vr=-600 V  diode_Ls=150 nH  diode_Erec=0.03 J  diode_rec_loss_model=ee.enum.diode.reverseRecoveryModel.fixed  diode_ErecVal=0 J  diode_scaleWithIandV=true  diode_ErecMat=zeros(2, 3) J  diode_TjrecVec=[298.15, 398.15] K  diode_IfrecVec=[.1, 1, 10] A  diode_IrecVal=10 A  diode_VrecVal=10 V  diode_tFilter=1 / 1000 / 100 s  thermal_network_parameterization=ee.enum.thermalNetworkTopology.external  Rth=[.03, .2] K/W  Rth_Cauer=[.03, .1, .2] K/W  Rth_Foster=[.03, .2] K/W  thermal_mass_parameterization=ee.enum.thermalNetwork.timeconstant  thermal_mass=[3, 25] J/K  thermal_mass_Cauer=[3, 10, 25] J/K  thermal_mass_Foster=[33, 50] J/K  thermal_time_constant=[.1, 5] s  thermal_time_constant_Cauer=[.1, 1, 5] s  thermal_time_constant_Foster=[1, 10] s  thermal_mass_initial_temperatures=[25, 25] degC  thermal_mass_initial_temperatures_Cauer=[25, 25, 25] degC  junction_thermal_mass=0.1 J/K  Tvec_initial_Foster=[25, 25, 25, 25] degC  no_thermal_network=0  junction_temperature_specify=off  junction_temperature_priority=None  junction_temperature=25 degC  junction_temperature_nominal_specify=off  junction_temperature_nominal_unit=degC  junction_temperature_nominal_value=1  Qj_specify=off  Qj_priority=None  Qj=0 W  Qj_nominal_specify=off  Qj_nominal_unit=W  Qj_nominal_value=1  accumulatedSwitchingLosses_specify=off  accumulatedSwitchingLosses_priority=None  accumulatedSwitchingLosses=0 J
  PGND : fl_lib/Electrical/Electrical Elements/Electrical Reference
  Rshunt : fl_lib/Electrical/Electrical Elements/Resistor  R=1 Ohm  i_specify=off  i_priority=None  i=0 A  i_nominal_specify=off  i_nominal_unit=A  i_nominal_value=1  v_specify=off  v_priority=None  v=0 V  v_nominal_specify=off  v_nominal_unit=V  v_nominal_value=1
  Scope1 : Scope  Commented=on  NumInputPorts=4
  Simulink-PS Converter{,1..3} (4 alike) : nesl_utility/Simulink-PS Converter  PhysicalDomain=network_engine_domain  SubClassName=ps_input  LeftPortType=input  RightPortType=output  PseudoPeriodic=off  Frequencies=[]  NoiseDistribution=none  NoiseParameters=[]  Unit=1  AffineConversion=off  FilteringAndDerivatives=provide  SimscapeFilterOrder=1  InputFilterTimeConstant=0.001  UdotUserProvided=0
  Subsystem : Subsystem
  Vin+ : PMIOPort  Side=Right
  Vin- : PMIOPort  Port=2  Side=Right
  Vpole+ : PMIOPort  Port=3  Side=Left
  Vpole- : PMIOPort  Port=4  Side=Left
  wires:
  [PWM3] -> Gain1/1
  [PWM1] -> Gain/1
  [PWM4] -> Gain3/1
  [PWM2] -> Gain2/1
  Gain/1 -> Simulink-PS Converter/1, Scope1/1
  Gain1/1 -> Simulink-PS Converter3/1, Scope1/3
  Gain2/1 -> Simulink-PS Converter1/1, Scope1/2
  Gain3/1 -> Scope1/4, Simulink-PS Converter2/1
  connections:
  Vin-/RConn1 -- "MOSFET (Ideal, Switching)4"/RConn2 -- PGND/LConn1 -- "MOSFET (Ideal, Switching)3"/RConn2
  "MOSFET (Ideal, Switching)"/RConn2 -- "MOSFET (Ideal, Switching)4"/RConn1 -- Subsystem/LConn1 -- Rshunt/LConn1
  Simulink-PS Converter3/RConn1 -- "MOSFET (Ideal, Switching)1"/LConn1
  "MOSFET (Ideal, Switching)3"/RConn1 -- Vpole-/RConn1 -- "MOSFET (Ideal, Switching)1"/RConn2
  "MOSFET (Ideal, Switching)1"/RConn1 -- Vin+/RConn1 -- "MOSFET (Ideal, Switching)"/RConn1
  "MOSFET (Ideal, Switching)4"/LConn1 -- Simulink-PS Converter1/RConn1
  Simulink-PS Converter2/RConn1 -- "MOSFET (Ideal, Switching)3"/LConn1
  Simulink-PS Converter/RConn1 -- "MOSFET (Ideal, Switching)"/LConn1
  Vpole+/RConn1 -- Subsystem/LConn2 -- Rshunt/RConn1

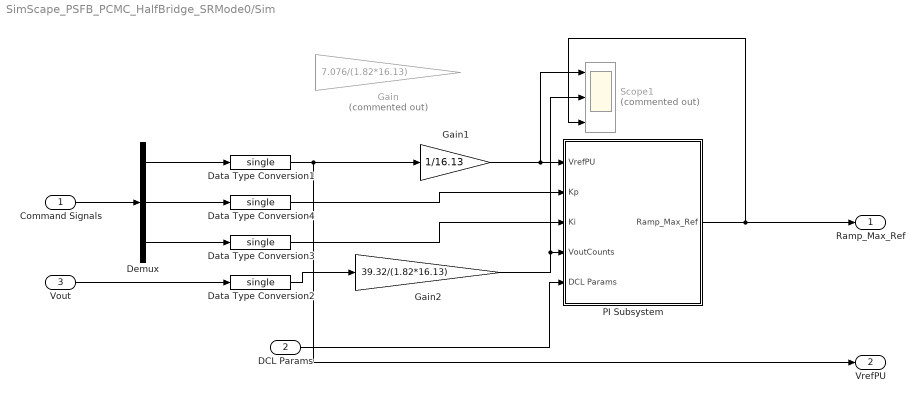
== system SimScape_PSFB_PCMC_HalfBridge_SRMode0/Sim ==
  Command Signals : Inport
  DCL Params : Inport  Port=2
  Vout : Inport  Port=3
  Data Type Conversion{1..4} (4 alike) : DataTypeConversion  OutDataTypeStr=single  SaturateOnIntegerOverflow=off  RndMeth=Floor
  Demux : Demux  Outputs=3
  Gain : Gain  Commented=on  Gain=7.076/(1.82*16.13)
  Gain1 : Gain  Gain=1/16.13  OutDataTypeStr=single
  Gain2 : Gain  Gain=39.32/(1.82*16.13)  OutDataTypeStr=single
  PI Subsystem : Subsystem
  Scope1 : Scope  Commented=on  NumInputPorts=3
  Ramp_Max_Ref : Outport
  VrefPU : Outport  Port=2
  wires:
  Demux/1 -> Data Type Conversion1/1
  Demux/3 -> Data Type Conversion3/1
  PI Subsystem/1(Ramp_Max_Ref) -> Scope1/3, Ramp_Max_Ref/1
  Demux/2 -> Data Type Conversion4/1
  Vout/1 -> Data Type Conversion2/1
  Command Signals/1 -> Demux/1
  Data Type Conversion3/1 -> PI Subsystem/3(Ki)
  Data Type Conversion4/1 -> PI Subsystem/2(Kp)
  DCL Params/1 -> PI Subsystem/5(DCL Params)
  Data Type Conversion1/1 -> Gain1/1, VrefPU/1
  Data Type Conversion2/1 -> Gain2/1
  Gain1/1 -> Scope1/1, PI Subsystem/1(VrefPU)
  Gain2/1 -> Scope1/2, PI Subsystem/4(VoutCounts)

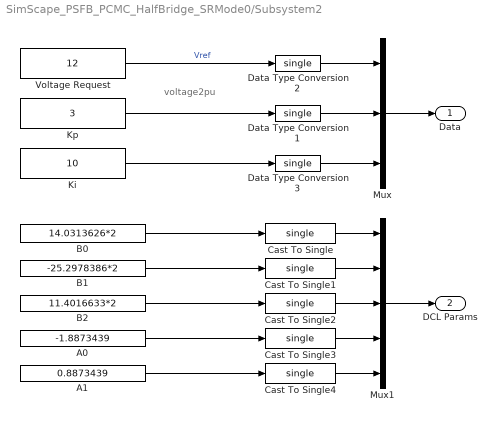
== system SimScape_PSFB_PCMC_HalfBridge_SRMode0/Subsystem2 ==
  note: voltage2pu
  A0 : Constant  Value=-1.8873439
  A1 : Constant  Value=0.8873439
  B0 : Constant  Value=14.0313626*2
  B1 : Constant  Value=-25.2978386*2
  B2 : Constant  Value=11.4016633*2
  Cast To Single{,1..4} (5 alike) : DataTypeConversion  OutDataTypeStr=single  SaturateOnIntegerOverflow=off  RndMeth=Floor
  Data Type Conversion1 : DataTypeConversion  OutDataTypeStr=single  RndMeth=Simplest  SaturateOnIntegerOverflow=off
      settings: AttributesFormatString=DataType = %<OutDataTypeStr>
  Data Type Conversion2 : DataTypeConversion  OutDataTypeStr=single  RndMeth=Simplest  SaturateOnIntegerOverflow=off
      settings: AttributesFormatString=DataType = %<OutDataTypeStr>
  Data Type Conversion3 : DataTypeConversion  OutDataTypeStr=single  RndMeth=Simplest  SaturateOnIntegerOverflow=off
      settings: AttributesFormatString=DataType = %<OutDataTypeStr>
  Ki : Constant  Value=10  SampleTime=-1
  Kp : Constant  Value=3  SampleTime=-1
  Mux : Mux  Inputs=3
  Mux1 : Mux  Inputs=5
  Voltage Request : Constant  Value=12  OutDataTypeStr=single  SampleTime=-1
  Data : Outport
  DCL Params : Outport  Port=2
  wires:
  Data Type Conversion1/1 -> Mux/2
  Ki/1 -> Data Type Conversion3/1
  Data Type Conversion2/1 -> Mux/1
  Kp/1 -> Data Type Conversion1/1
  Voltage Request/1 -> Data Type Conversion2/1  "Vref"
  Data Type Conversion3/1 -> Mux/3
  Mux/1 -> Data/1
  B0/1 -> Cast To Single/1
  B1/1 -> Cast To Single1/1
  A1/1 -> Cast To Single4/1
  Cast To Single/1 -> Mux1/1
  Cast To Single1/1 -> Mux1/2
  Cast To Single2/1 -> Mux1/3
  B2/1 -> Cast To Single2/1
  Cast To Single3/1 -> Mux1/4
  A0/1 -> Cast To Single3/1
  Cast To Single4/1 -> Mux1/5
  Mux1/1 -> DCL Params/1

== system SimScape_PSFB_PCMC_HalfBridge_SRMode0/Comparator/DEC Counts ==
  note: 3.3 / (1/16.13)
  VrefPU : Inport
  Constant : Constant  Value=ADC_MaxCount*Tcmpss*Gi_fb/(ADC_Vref*L*2)  VectorParams1D=off
  Gain : Gain  Gain=1/3.3
  Product : Product
  DEC : Outport
  wires:
  Constant/1 -> Product/2
  VrefPU/1 -> Gain/1
  Product/1 -> DEC/1
  Gain/1 -> Product/1

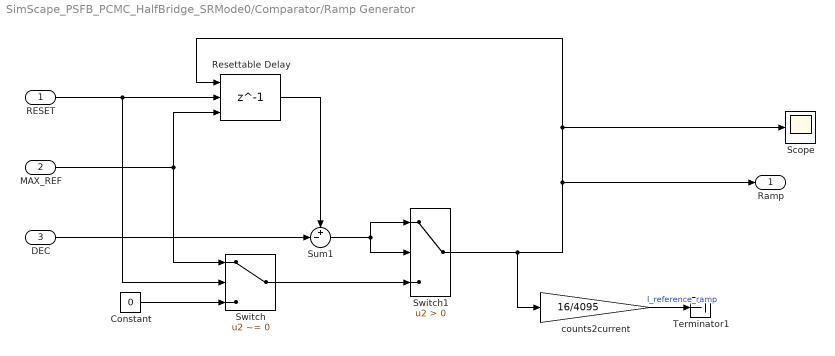
== system SimScape_PSFB_PCMC_HalfBridge_SRMode0/Comparator/Ramp Generator ==
  RESET : Inport
  MAX_REF : Inport  Port=2
  DEC : Inport  Port=3
  Constant : Constant  Value=0
  Resettable Delay : Delay  DelayLength=1  InitialConditionSource=Input port  ExternalReset=Rising
      settings: InputPortMap=u0,r5,p4
  Scope : Scope
  Sum1 : Sum  Inputs=+-|
  Switch : Switch  Criteria=u2 ~= 0  SaturateOnIntegerOverflow=off  InputSameDT=off
  Switch1 : Switch  Criteria=u2 > Threshold  SaturateOnIntegerOverflow=off  InputSameDT=off
  Terminator1 : Terminator
  counts2current : Gain  Gain=16/4095
  Ramp : Outport
  wires:
  MAX_REF/1 -> Switch/1, Resettable Delay/3
  Switch1/1 -> counts2current/1, Ramp/1, Scope/1, Resettable Delay/1
  RESET/1 -> Switch/2, Resettable Delay/2
  Sum1/1 -> Switch1/1, Switch1/2
  DEC/1 -> Sum1/2
  Resettable Delay/1 -> Sum1/1
  Constant/1 -> Switch/3
  counts2current/1 -> Terminator1/1  "I_reference_ramp"
  Switch/1 -> Switch1/3

== system SimScape_PSFB_PCMC_HalfBridge_SRMode0/Load/Voltage Sensing ==
  note: Scaling factor
      | Vsense = Vo * (1.82/39.32)
  PS-Simulink Converter : nesl_utility/PS-Simulink Converter  PhysicalDomain=network_engine_domain  SubClassName=ps_output  LeftPortType=input  RightPortType=output  PseudoPeriodic=off  Frequencies=[]  VectorFormat=inherit  Unit=inherit  AffineConversion=off
  R1 : fl_lib/Electrical/Electrical Elements/Resistor  R=1.82e3 Ohm  i_specify=off  i_priority=None  i=0 A  i_nominal_specify=off  i_nominal_unit=A  i_nominal_value=1  v_specify=off  v_priority=None  v=0 V  v_nominal_specify=off  v_nominal_unit=V  v_nominal_value=1
  R2 : fl_lib/Electrical/Electrical Elements/Resistor  R=37.593e3 Ohm  i_specify=off  i_priority=None  i=0 A  i_nominal_specify=off  i_nominal_unit=A  i_nominal_value=1  v_specify=off  v_priority=None  v=0 V  v_nominal_specify=off  v_nominal_unit=V  v_nominal_value=1
  Voltage Sensor : fl_lib/Electrical/Electrical Sensors/Voltage Sensor
  In+ : PMIOPort  Side=Left
  In- : PMIOPort  Port=2  Side=Left
  tag scope: Vout=global
  wires:
  PS-Simulink Converter/1 -> [Vout]
  connections:
  R2/RConn1 -- Voltage Sensor/LConn1 -- R1/LConn1
  R1/RConn1 -- Voltage Sensor/RConn2 -- In-/RConn1
  In+/RConn1 -- R2/LConn1
  Voltage Sensor/RConn1 -- PS-Simulink Converter/LConn1

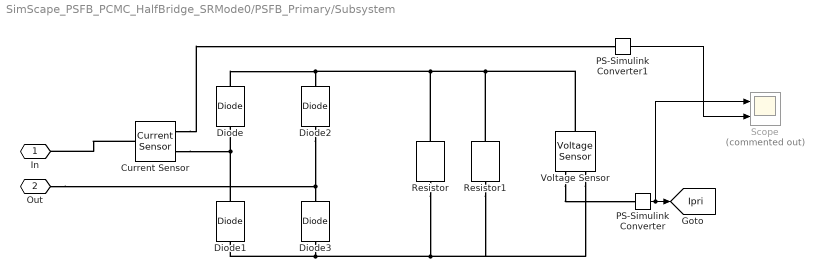
== system SimScape_PSFB_PCMC_HalfBridge_SRMode0/PSFB_Primary/Subsystem ==
  Current Sensor : fl_lib/Electrical/Electrical Sensors/Current Sensor
  Diode{,1..3} (4 alike) : ee_lib/Semiconductors & Converters/Diode  ModelType=ee.enum.diode.modelType.pwl  TableType=ee.enum.diode.tableType.IfMat  IfMat=[.07, .12, .19, 1.75, 4.24, 7.32, 11.2; .16, .3, .72, 2.14, 5.02, 8.35, 13.12] A  VfMat=[.9, 1.15, 1.25, 1.5, 1.75, 2.17, 2.6, 2.85; .58, .68, .75, 1.1, 1.38, 1.77, 2.27, 2.7] V  TjVec=[25, 125] degC  VfVec=[.5, .7, .9, 1.3, 1.7, 2.1, 2.5] V  IfVec=[.1, .2, .5, 1, 2, 4, 7, 10] A  Vf=0.6 V  Ron=0.3e-6 Ohm  Goff=1e-8 S  prmExp=ee.enum.diode.expParam.useTwo  I12=[.0137, .545] A  V12=[.6, .7] V  RS=0 Ohm  Tmeas=25 degC  IS=1e-12 A  ec=1  I1=0.0137 A  V1=0.6 V  N_series=1  N_parallel=1  ZenerEnable=false  Rz=0.3 Ohm  BV=inf V  C_param=ee.enum.diode.capParam.fixed  CJ=0 pF  CJ0=5 pF  Vvec=[.1, 10, 100] V  Cvec=[3.5, 1, .4] pF  VJ=1 V  Mgrad=0.5  FC=0.5  Q_param=ee.enum.diode.recoveryParam.off  iRM=-7.15 A  iF=4 A  didt=-750 A/us  trr_factor=3  trr=115 ns  Qrr=150 nA*s  Vr=-600 V  Ls=150 nH  Erec=0.03 J  TT=50 ns  tau=100 ns  T_param=ee.enum.diode.temperatureParam.off  Tdevice=25 degC  I1_T2=0.245 A  V1_T2=0.5 V  IS_T2=1.25e-7 A  Tmeas2=125 degC  XTI_param=ee.enum.diode.xtiParam.pn  XTI=3  EG_param=ee.enum.diode.egapParam.material_si  EG=1.11 eV  dBVdT=0 V/K  enable_faults=simscape.enum.onoff.off  fault_action=simscape.enum.assert.action.none  fault_types=ee.enum.diode.faults.open  tau_fault=1e-3 s  IfMat_faulted=[.07, .12, .19, 1.75, 4.24, 7.32, 11.2; .16, .3, .72, 2.14, 4.02, 6.35, 9.12] A  VfMat_faulted=[.9, 1.15, 1.25, 1.5, 1.75, 2.17, 2.6, 2.85; .58, .68, .75, 1.1, 1.38, 1.77, 2.27, 2.7] V  VfVec_faulted=[.5, .7, .9, 1.3, 1.7, 2.1, 2.5] V  IfVec_faulted=[.1, .2, .5, 1, 2, 4, 7, 10] A  Ropen_faulted=1000 Ohm  Gshort_faulted=1000 1/Ohm  Vf_faulted=0.6 V  Ron_faulted=0.3 Ohm  Goff_faulted=1e-8 S  I12_faulted=[.0137, .545] A  V12_faulted=[.6, .7] V  IS_faulted=1e-12 A  ec_faulted=1  I1_faulted=0.0137 A  V1_faulted=0.6 V  RS_faulted=0 Ohm  Rz_faulted=0.3 Ohm  BV_faulted=inf V  Cscale_faulted=100  fault_trigger=ee.enum.faults.faultTrigger.temporal  t_fault=inf s  max_permissible_voltage=inf V  n_fail_on_voltage=1  max_permissible_current=inf A  t_fail_on_current=1 s  max_permissible_dVdt=inf V/s  enable_fault_input=simscape.enum.onoff.off  i_specify=off  i_priority=None  i=0 A  i_nominal_specify=off  i_nominal_unit=A  i_nominal_value=1  v_specify=off  v_priority=None  v=0 V  v_nominal_specify=off  v_nominal_unit=V  v_nominal_value=1  v_capacitor_specify=off  v_capacitor_priority=None  v_capacitor=0 V  v_capacitor_nominal_specify=off  v_capacitor_nominal_unit=V  v_capacitor_nominal_value=1  faulted_specify=off  faulted_priority=None  faulted=0  faulted_nominal_specify=off  faulted_nominal_unit=1  faulted_nominal_value=1  i_diode_specify=off  i_diode_priority=None  i_diode=0 A  i_diode_nominal_specify=off  i_diode_nominal_unit=A  i_diode_nominal_value=1  v_diode_specify=off  v_diode_priority=None  v_diode=0 V  v_diode_nominal_specify=off  v_diode_nominal_unit=V  v_diode_nominal_value=1  i_capacitor_specify=off  i_capacitor_priority=None  i_capacitor=0 A  i_capacitor_nominal_specify=off  i_capacitor_nominal_unit=A  i_capacitor_nominal_value=1  power_dissipated_specify=off  power_dissipated_priority=None  power_dissipated=0 W  power_dissipated_nominal_specify=off  power_dissipated_nominal_unit=W  power_dissipated_nominal_value=1  fidelity_level=ee.enum.diode.fidelity.includeChargeDyn  rec_loss_model=ee.enum.diode.reverseRecoveryModel.fixed  ErecVal=0 J  scaleWithIandV=true  ErecMat=zeros(2, 3) J  TjrecVec=[298.15, 398.15] K  IfrecVec=[.1, 1, 10] A  IrecVal=10 A  VrecVal=10 V  tFilter=1 / 1000 / 100 s  max_permissible_temperature=inf K  t_fail_on_temperature=1 s  thermal_network_parameterization=ee.enum.thermalNetworkTopology.junctionCase  Rth=[0, 10] K/W  Rth_Cauer=[1, 3, 10] K/W  Rth_Foster=[4, 6] K/W  thermal_mass_parameterization=ee.enum.thermalNetwork.timeconstant  thermal_mass=[0, 1] J/K  thermal_mass_Cauer=[.1, .3, 1] J/K  thermal_mass_Foster=[1.5, 3] J/K  thermal_time_constant=[0, 10] s  thermal_time_constant_Cauer=[1, 3, 10] s  thermal_time_constant_Foster=[6, 18] s  thermal_mass_initial_temperatures=[25, 25] degC  thermal_mass_initial_temperatures_Cauer=[25, 25, 25] degC  junction_thermal_mass=0.01 J/K  Tvec_initial_Foster=[25, 25, 25, 25] degC  no_thermal_network=0  junction_temperature_specify=off  junction_temperature_priority=None  junction_temperature=25 degC  junction_temperature_nominal_specify=off  junction_temperature_nominal_unit=degC  junction_temperature_nominal_value=1
  PS-Simulink Converter : nesl_utility/PS-Simulink Converter  PhysicalDomain=network_engine_domain  SubClassName=ps_output  LeftPortType=input  RightPortType=output  PseudoPeriodic=off  Frequencies=[]  VectorFormat=inherit  Unit=inherit  AffineConversion=off
  PS-Simulink Converter1 : nesl_utility/PS-Simulink Converter  PhysicalDomain=network_engine_domain  SubClassName=ps_output  LeftPortType=input  RightPortType=output  PseudoPeriodic=off  Frequencies=[]  VectorFormat=inherit  Unit=inherit  AffineConversion=off
  Resistor : fl_lib/Electrical/Electrical Elements/Resistor  R=9.72e3 Ohm  i_specify=off  i_priority=None  i=0 A  i_nominal_specify=off  i_nominal_unit=A  i_nominal_value=1  v_specify=off  v_priority=None  v=0 V  v_nominal_specify=off  v_nominal_unit=V  v_nominal_value=1
  Resistor1 : fl_lib/Electrical/Electrical Elements/Resistor  R=14.7/2 Ohm  i_specify=off  i_priority=None  i=0 A  i_nominal_specify=off  i_nominal_unit=A  i_nominal_value=1  v_specify=off  v_priority=None  v=0 V  v_nominal_specify=off  v_nominal_unit=V  v_nominal_value=1
  Scope : Scope  Commented=on  NumInputPorts=2
  Voltage Sensor : fl_lib/Electrical/Electrical Sensors/Voltage Sensor
  In : PMIOPort  Side=Left
  Out : PMIOPort  Port=2  Side=Left
  tag scope: Ipri=global
  wires:
  PS-Simulink Converter/1 -> Scope/1, [Ipri]
  PS-Simulink Converter1/1 -> Scope/2
  connections:
  Voltage Sensor/LConn1 -- Resistor1/LConn1 -- Resistor/LConn1 -- Diode/RConn1 -- Diode2/RConn1
  Diode3/LConn1 -- Resistor/RConn1 -- Resistor1/RConn1 -- Voltage Sensor/RConn2 -- Diode1/LConn1
  Diode1/RConn1 -- Diode/LConn1 -- Current Sensor/RConn2
  Diode2/LConn1 -- Out/RConn1 -- Diode3/RConn1
  Voltage Sensor/RConn1 -- PS-Simulink Converter/LConn1
  Current Sensor/LConn1 -- In/RConn1
  Current Sensor/RConn1 -- PS-Simulink Converter1/LConn1

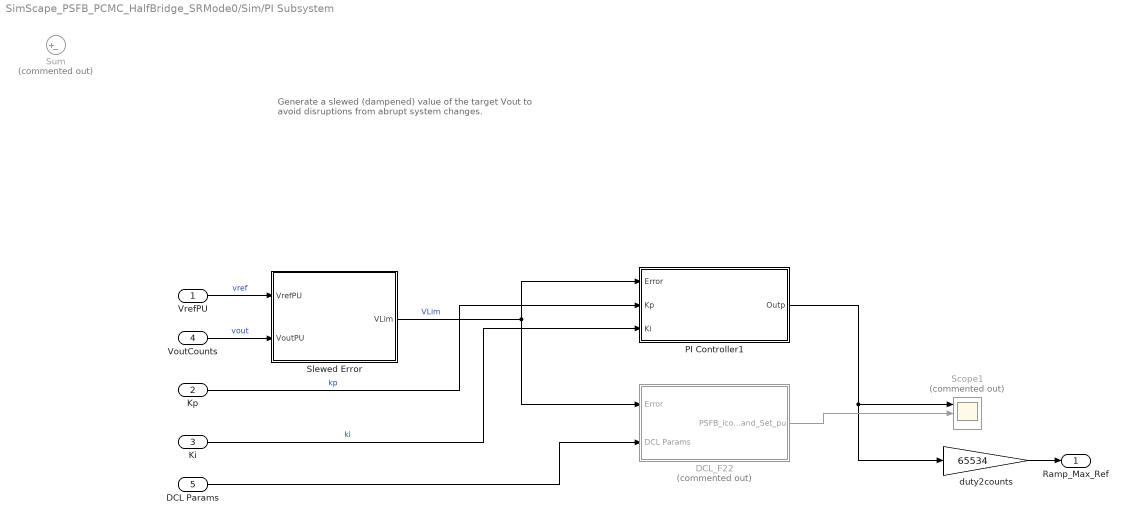
== system SimScape_PSFB_PCMC_HalfBridge_SRMode0/Sim/PI Subsystem ==
  note: Generate a slewed (dampened) value of the target Vout to avoid disruptions from abrupt system changes.
  VrefPU : Inport  OutDataTypeStr=single
  Kp : Inport  Port=2  OutDataTypeStr=single
  Ki : Inport  Port=3  OutDataTypeStr=single
  VoutCounts : Inport  Port=4  OutDataTypeStr=single
  DCL Params : Inport  Port=5
  DCL_F22 : Subsystem  Commented=on
  PI Controller1 : Subsystem
  Scope1 : Scope  Commented=on  NumInputPorts=3
  Slewed Error : Subsystem
  Sum : Sum  Commented=on  Inputs=|+-
  duty2counts : Gain  Gain=65534  OutDataTypeStr=single
  Ramp_Max_Ref : Outport
  wires:
  Slewed Error/1(VLim) -> PI Controller1/1(Error), DCL_F22/1(Error)  "VLim"
  VrefPU/1 -> Slewed Error/1(VrefPU)  "vref"
  VoutCounts/1 -> Slewed Error/2(VoutPU)  "vout"
  Ki/1 -> PI Controller1/3(Ki)  "ki"
  Kp/1 -> PI Controller1/2(Kp)  "kp"
  duty2counts/1 -> Ramp_Max_Ref/1
  DCL Params/1 -> DCL_F22/2(DCL Params)
  PI Controller1/1(Outp) -> duty2counts/1, Scope1/1
  DCL_F22/1(PSFB_icommand_Set_pu) -> Scope1/2

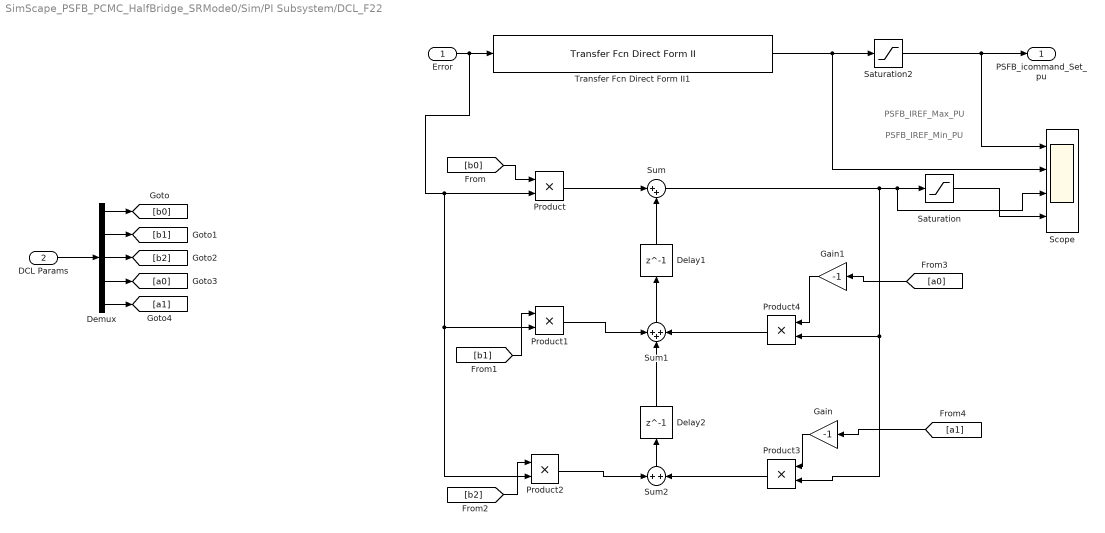
== system SimScape_PSFB_PCMC_HalfBridge_SRMode0/Sim/PI Subsystem/DCL_F22 ==
  note: PSFB_IREF_Min_PU
  note: PSFB_IREF_Max_PU
  Error : Inport
  DCL Params : Inport  Port=2
  Delay1 : Delay  DelayLength=1
  Delay2 : Delay  DelayLength=1
  Demux : Demux  Outputs=5
  Gain : Gain  Gain=-1
  Gain1 : Gain  Gain=-1
  Product{,1..4} (5 alike) : Product
  Saturation : Saturate  UpperLimit=0.9  LowerLimit=0.06
  Saturation2 : Saturate  UpperLimit=0.9  LowerLimit=0.06
  Scope : Scope  NumInputPorts=4
  Sum : Sum  Inputs=|++
  Sum1 : Sum  Inputs=+++
  Sum2 : Sum  Inputs=+|+
  Transfer Fcn Direct Form II1 : simulink/Additional Math & Discrete/Additional Discrete/Transfer Fcn Direct Form II  NumCoefVec=[14.0213636*2 -25.2978386*2 11.4016633*2]  DenCoefVec=[-1.8873439 0.8873439]  vinit=0.0  DoSatur=off
  PSFB_icommand_Set_pu : Outport
  wires:
  Delay1/1 -> Sum/2
  Delay2/1 -> Sum1/2
  Product3/1 -> Sum2/2
  Error/1 -> Product/2, Product2/2, Product1/2, Transfer Fcn Direct Form II1/1
  Product1/1 -> Sum1/1
  Sum2/1 -> Delay2/1
  Product/1 -> Sum/1
  Sum1/1 -> Delay1/1
  Product2/1 -> Sum2/1
  Product4/1 -> Sum1/3
  DCL Params/1 -> Demux/1
  Demux/1 -> [b0]
  Demux/5 -> [a1]
  Demux/4 -> [a0]
  Demux/3 -> [b2]
  Demux/2 -> [b1]
  [b0] -> Product/1
  [b2] -> Product2/1
  [b1] -> Product1/1
  Gain/1 -> Product3/1
  [a1] -> Gain/1
  Gain1/1 -> Product4/1
  [a0] -> Gain1/1
  Sum/1 -> Product4/2, Product3/2, Scope/3, Saturation/1
  Transfer Fcn Direct Form II1/1 -> Scope/2, Saturation2/1
  Saturation2/1 -> Scope/1, PSFB_icommand_Set_pu/1
  Saturation/1 -> Scope/4
